simulink model "PID_theory"  (R2015a)
settings: Solver=ode3  SolverMode=SingleTasking  StartTime=0.0  StopTime=20  FixedStep=0.001  RelTol=1e-3
settings Model: CovMetricSettings=dwe  CovHtmlReporting=off  covSaveCumulativeToWorkspaceVar=off  CovSaveSingleToWorkspaceVar=off  CovExternalEMLEnable=on  Creator=DwigHT  LastModifiedBy=DwigHT
settings DataIOCC: LimitDataPoints=off  SaveFormat=Dataset  ReturnWorkspaceOutputs=on
settings DebuggingCC: UnconnectedInputMsg=none  UnconnectedOutputMsg=none  UnconnectedLineMsg=none  SFUnexpectedBacktrackingDiag=error  SFNoUnconditionalDefaultTransitionDiag=error
settings HardwareCC: ProdBitPerPointer=64  ProdLargestAtomicFloat=Float  ProdIntDivRoundTo=Zero  ProdEndianess=LittleEndian  ProdHWDeviceType=Specified
settings ModelReferenceCC: PropagateSignalLabelsOutOfModel=on
settings SFSimCC: SimUseLocalCustomCode=on
settings RTWCC: RTWUseLocalCustomCode=on
settings GRTTargetCC: TargetLangStandard=C99 (ISO)

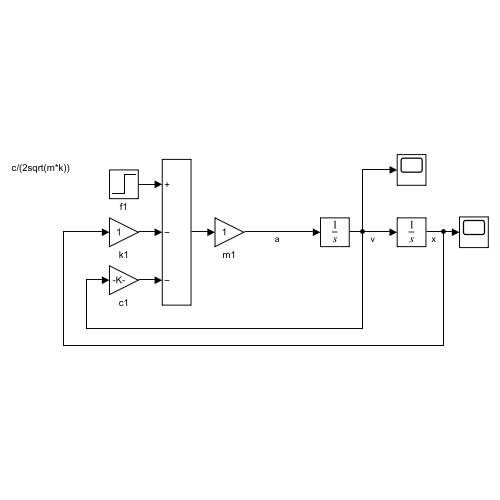
[thumbnail: Simulink's stored preview of the top-level diagram]
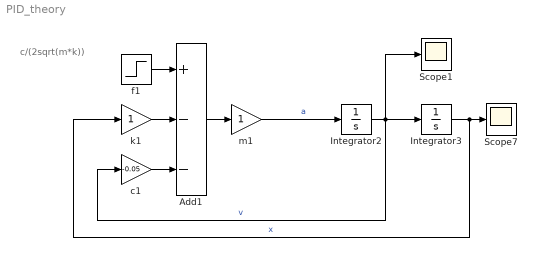
== system PID_theory ==
  note: c/(2sqrt(m*k))
  Add1 : Sum  Inputs=+--
  Integrator2 : Integrator
  Integrator3 : Integrator
  Scope1 : Scope
      settings: TimeRange=auto  MaxDataPoints=5000  SaveToWorkspace=off  YMin=-1.91226  YMax=1.7958  SampleTime=-1
  Scope7 : Scope
      settings: TimeRange=auto  MaxDataPoints=5000  SaveToWorkspace=off  YMin=-0.98763  YMax=2.86658  SampleTime=-1
  c1 : Gain  Gain=-0.05
  f1 : Step  SampleTime=0
  k1 : Gain
  m1 : Gain
  wires:
  f1/1 -> Add1/1
  Integrator3/1 -> Scope7/1, k1/1  "x"
  c1/1 -> Add1/3
  k1/1 -> Add1/2
  Integrator2/1 -> Scope1/1, Integrator3/1, c1/1  "v"
  m1/1 -> Integrator2/1  "a"
  Add1/1 -> m1/1
